simulink model "buck_04_2018_b"  (Simulink 9.2)
settings: Solver=ode45  StartTime=0.0  StopTime=1000/F  MaxStep=1/(10*F)  RelTol=1e-3  EnableMultiTasking=on
values from neighbouring files (symbols this model uses):
  C = 9.3e-6    (= 9.3e-06)    [buck_01_script.m]    (also in buck_02_script.m; buck_04_script.m)
  C1 = 5.5e-6    (= 5.5e-06)    [buck_01_script.m]    (also in buck_02_script.m; buck_04_script.m)
  duty = Vs / Ve    (= 0.66)    [buck_01_script.m]    (also in buck_02_script.m; buck_04_script.m)
  L = 1.9e-6    (= 1.9e-06)    [buck_01_script.m]    (also in buck_02_script.m; buck_04_script.m)
  L1 = 5e-6    (= 5e-06)    [buck_01_script.m]    (also in buck_02_script.m; buck_04_script.m)
  R = Vs^2 / Ps    (= 5.445)    [buck_01_script.m]    (also in buck_02_script.m = 0.5445; buck_04_script.m)
  Ve = 5    [buck_01_script.m]    (also in buck_02_script.m; buck_04_script.m)
libraries: powerlib x14
settings Model: Creator=lefrancp  LastModifiedBy=lefrancp
settings DataIOCC: SaveFinalState=on  SignalLoggingSaveFormat=Dataset  SaveOutput=off
settings DebuggingCC: UnderspecifiedInitializationDetection=Simplified  MergeDetectMultiDrivingBlocksExec=error  SolverPrmCheckMsg=warning  FcnCallInpInsideContextMsg=error  StateNameClashWarn=none
settings GRTTargetCC: CombineOutputUpdateFcns=on  GRTInterface=off
settings ConfigComp: CovSFcnEnable=off
settings SimscapeCC: SimscapeNormalizeSystem=off

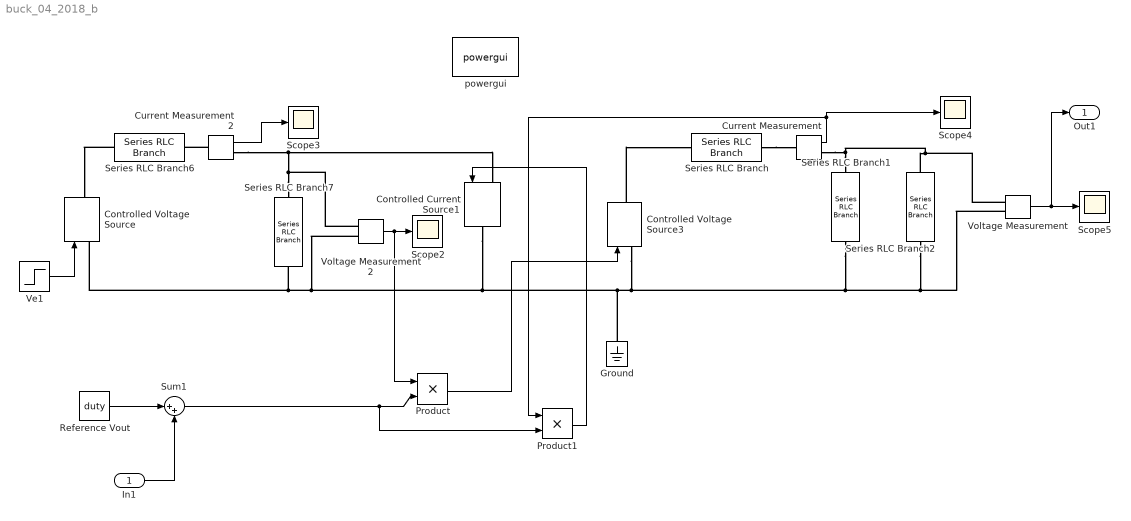
== system buck_04_2018_b ==
  In1 : Inport
  Controlled Current Source1 : powerlib/Electrical Sources/Controlled Current Source  Initialize=on  Source_Type=AC  Amplitude=0  Phase=0  Frequency=0  Measurements=None
  Controlled Voltage Source : powerlib/Electrical Sources/Controlled Voltage Source  Initialize=on  Source_Type=AC  Amplitude=0  Phase=0  Frequency=0  Measurements=None
  Controlled Voltage Source3 : powerlib/Electrical Sources/Controlled Voltage Source  Initialize=on  Source_Type=AC  Amplitude=0  Phase=0  Frequency=0  Measurements=None
  Current Measurement : powerlib/Measurements/Current Measurement  PhasorSimulation=off  OutputType=Complex  PSBequivalent=0
  Current Measurement2 : powerlib/Measurements/Current Measurement  PhasorSimulation=off  OutputType=Complex  PSBequivalent=0
  Ground : powerlib/Elements/Ground  LConnTagsString=a
  Product : Product
  Product1 : Product
  Reference Vout : Constant  Value=duty
  Scope{2..5} (4 alike) : Scope
  Series RLC Branch : powerlib/Elements/Series RLC Branch  LConnTagsString=__new0  RConnTagsString=__new0  BranchType=L  Resistance=1  Inductance=L  SetiL0=off  InitialCurrent=0  Capacitance=1e-6  Setx0=off  InitialVoltage=0  Measurements=None
  Series RLC Branch1 : powerlib/Elements/Series RLC Branch  LConnTagsString=__new0  RConnTagsString=__new0  BranchType=C  Resistance=1  Inductance=L  SetiL0=off  InitialCurrent=0  Capacitance=C  Setx0=off  InitialVoltage=0  Measurements=None
  Series RLC Branch2 : powerlib/Elements/Series RLC Branch  LConnTagsString=__new0  RConnTagsString=__new0  BranchType=R  Resistance=R  Inductance=L  SetiL0=off  InitialCurrent=0  Capacitance=C  Setx0=off  InitialVoltage=0  Measurements=None
  Series RLC Branch6 : powerlib/Elements/Series RLC Branch  LConnTagsString=__new0  RConnTagsString=__new0  BranchType=L  Resistance=1  Inductance=L1  SetiL0=off  InitialCurrent=0  Capacitance=1e-6  Setx0=off  InitialVoltage=0  Measurements=None
  Series RLC Branch7 : powerlib/Elements/Series RLC Branch  LConnTagsString=__new0  RConnTagsString=__new0  BranchType=C  Resistance=1  Inductance=L  SetiL0=off  InitialCurrent=0  Capacitance=C1  Setx0=off  InitialVoltage=0  Measurements=None
  Sum1 : Sum  Inputs=|++
  Ve1 : Step  Time=1e-4  Before=Ve  After=Ve  SampleTime=0
  Voltage Measurement : powerlib/Measurements/Voltage Measurement  PhasorSimulation=off  OutputType=Complex  PSBequivalent=0
  Voltage Measurement2 : powerlib/Measurements/Voltage Measurement  PhasorSimulation=off  OutputType=Complex  PSBequivalent=0
  powergui : powerlib/powergui  Priority=1  SimulationMode=Continuous  SampleTime=50e-6  frequency=60  Iterations=50  frequencyindice=0  Pbase=100e6  ErrMax=1e-4  UnitsV=kV  UnitsW=MW  buscounter=0  FunctionMessages=off  echomessages=off  EnableUseOfTLC=off  CurrentSourceSwitches=on  DisableSnubberDevices=off  DisableRonSwitches=off  DisableVfSwitches=off  DisplayEquations=off  AutomaticDiscreteSolvers=off  SolverType=Tustin  Interpol=off  ExternalGateDelay=off  methode=off  Ts=0  x0status=blocks  SPID=off  SwTol=0  HookPort=off  NonlinearTolerance=0  nMaxIteration=15  ContinueOnMaxIteration=off  RestoreLinks=warning  ResistiveCurrentMeasurement=off  Frange=[0:2:500]  Ylog=off  Xlog=on  ShowGrid=off  save=off  variable=ZData  structure=0  ZoomFFT=off  StartTime=0.0  cycles=1  DisplayStyle=1  fundamental=60  FreqAxis=off  MaxFrequency=1000  frequencyindicesteady=1  RmsSteady=1  display=off
  Out1 : Outport  VectorParamsAs1DForOutWhenUnconnected=off
  wires:
  Voltage Measurement/1 -> Out1/1, Scope5/1
  Current Measurement/1 -> Product1/1, Scope4/1
  Ve1/1 -> Controlled Voltage Source/1
  Voltage Measurement2/1 -> Product/1, Scope2/1
  Current Measurement2/1 -> Scope3/1
  Sum1/1 -> Product1/2, Product/2
  Product/1 -> Controlled Voltage Source3/1
  Product1/1 -> Controlled Current Source1/1
  Reference Vout/1 -> Sum1/1
  In1/1 -> Sum1/2
  connections:
  Ground/LConn1 -- Controlled Voltage Source3/LConn1 -- Series RLC Branch1/RConn1 -- Voltage Measurement/LConn2 -- Series RLC Branch2/RConn1 -- Controlled Current Source1/RConn1 -- Voltage Measurement2/LConn2 -- Series RLC Branch7/RConn1 -- Controlled Voltage Source/LConn1
  Controlled Voltage Source3/RConn1 -- Series RLC Branch/LConn1
  Series RLC Branch1/LConn1 -- Current Measurement/RConn1 -- Series RLC Branch2/LConn1 -- Voltage Measurement/LConn1
  Series RLC Branch7/LConn1 -- Voltage Measurement2/LConn1 -- Controlled Current Source1/LConn1 -- Current Measurement2/RConn1
  Series RLC Branch/RConn1 -- Current Measurement/LConn1
  Series RLC Branch6/LConn1 -- Controlled Voltage Source/RConn1
  Current Measurement2/LConn1 -- Series RLC Branch6/RConn1
